simulink library "fmCopterGuidedIndi_lib"  (R2018b)
settings: Solver=VariableStepAuto  StartTime=0.0  StopTime=10.0  RelTol=1e-3
undefined symbols (not defined in the file or in its folder): fm_Traj
libraries: traj_lib x1
settings Model: Creator=Ybeyer  LastModifiedBy=yannic
settings SFSimCC: SimUseLocalCustomCode=off
settings RTWCC: RTWUseLocalCustomCode=off
settings CodeAppCC: StateflowObjectComments=on

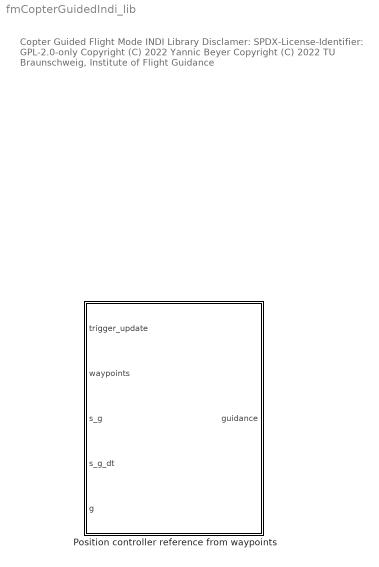
== system fmCopterGuidedIndi_lib ==
  note: Copter Guided Flight Mode INDI Library
      |
      | Disclamer:
      | SPDX-License-Identifier: GPL-2.0-only
      |
      | Copyright (C) 2022 Yannic Beyer
      | Copyright (C) 2022 TU Braunschweig, Institute of Flight Guidance
  Position controller reference from waypoints : Subsystem  mask{fm=fm_Traj, T_inner_loop=0.1}
      mask prompts: fm "Guided flight mode parameters struct, see fmCopterGuidedIndi_params_default"; T_inner_loop "Inner loop time constant seen by position controller, in s"
      mask init:
      | % Create emptry trajectory with a maximum space for 10 waypoints
      | [traj_empty] = trajInit(fm.traj.wpmax, fm.traj.degree);
      | 
      | % Create simulink bus definition
      | assignin('base','trajectoryBus', struct2bus_(traj_empty));
      mask DialogControl DescGroupVar Prompt: Position controller reference from waypoints
      mask DialogControl DescTextVar Prompt: Waypoints are connected by splines. The shortest distance to the desired flight path is computed. Then the corresponding desired position, velocity and acceleration are computed based on the desired flight-path velocity.

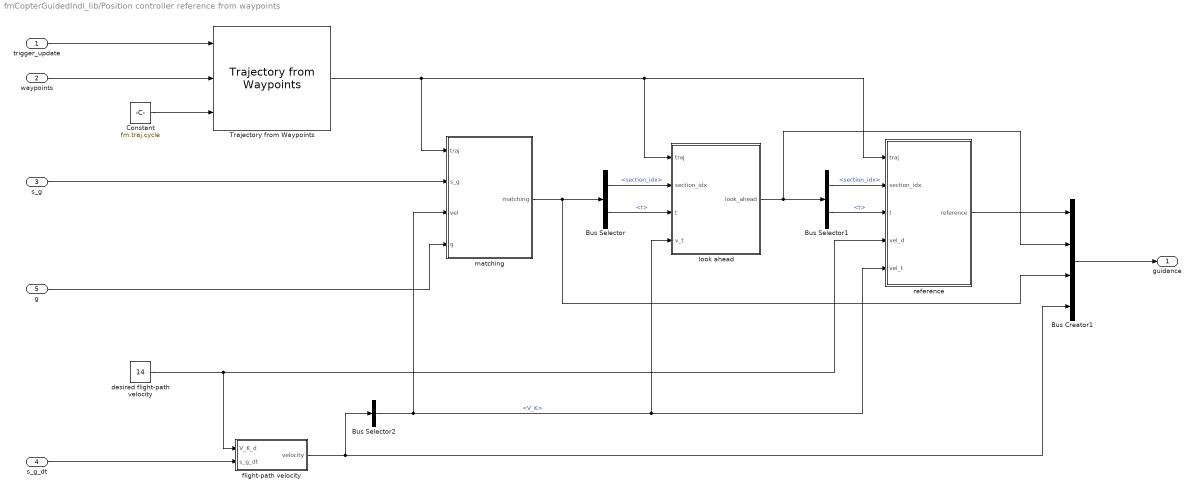
== system fmCopterGuidedIndi_lib/Position controller reference from waypoints ==
  trigger_update : Inport
  waypoints : Inport  Port=2
  s_g : Inport  Port=3
  s_g_dt : Inport  Port=4
  g : Inport  Port=5
  Bus Creator1 : BusCreator  Inputs=4
  Bus Selector : BusSelector  OutputSignals=section_idx,t
  Bus Selector1 : BusSelector  OutputSignals=section_idx,t
  Bus Selector2 : BusSelector  OutputSignals=V_K
  Constant : Constant  Value=fm.traj.cycle
  Trajectory from Waypoints : traj_lib/Trajectory from Waypoints  traj_empty=traj_empty
      settings: SourceProductName=LADAC
  desired flight-path velocity : Constant  Value=14
  flight-path velocity : Subsystem
  look ahead : Subsystem
  matching : Subsystem
  reference : Subsystem
  guidance : Outport
  wires:
  waypoints/1 -> Trajectory from Waypoints/2
  g/1 -> matching/4(g)
  Constant/1 -> Trajectory from Waypoints/3
  trigger_update/1 -> Trajectory from Waypoints/1
  Trajectory from Waypoints/1 -> look ahead/1(traj), reference/1(traj), matching/1(traj)
  s_g/1 -> matching/2(s_g)
  matching/1(matching) -> Bus Creator1/3, Bus Selector/1
  desired flight-path velocity/1 -> flight-path velocity/1(V_K_d), reference/4(vel_d)
  look ahead/1(look_ahead) -> Bus Creator1/2, Bus Selector1/1
  reference/1(reference) -> Bus Creator1/1
  Bus Selector/1 -> look ahead/2(section_idx)  "<section_idx>"
  Bus Selector/2 -> look ahead/3(t)  "<t>"
  Bus Selector1/1 -> reference/2(section_idx)  "<section_idx>"
  Bus Selector1/2 -> reference/3(t)  "<t>"
  Bus Creator1/1 -> guidance/1
  s_g_dt/1 -> flight-path velocity/2(s_g_dt)
  flight-path velocity/1(velocity) -> Bus Creator1/4, Bus Selector2/1
  Bus Selector2/1 -> matching/3(vel), reference/5(vel_t), look ahead/4(v_t)  "<V_K>"

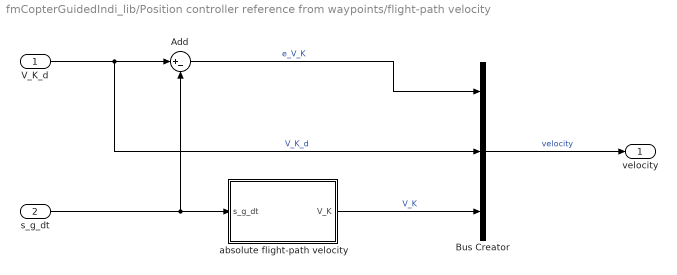
== system fmCopterGuidedIndi_lib/Position controller reference from waypoints/flight-path velocity ==
  V_K_d : Inport
  s_g_dt : Inport  Port=2
  Add : Sum  Inputs=|+-
  Bus Creator : BusCreator  Inputs=3
  absolute flight-path velocity : Subsystem
  velocity : Outport
  wires:
  s_g_dt/1 -> absolute flight-path velocity/1(s_g_dt), Add/2
  absolute flight-path velocity/1(V_K) -> Bus Creator/3  "V_K"
  V_K_d/1 -> Bus Creator/2, Add/1  "V_K_d"
  Bus Creator/1 -> velocity/1  "velocity"
  Add/1 -> Bus Creator/1  "e_V_K"

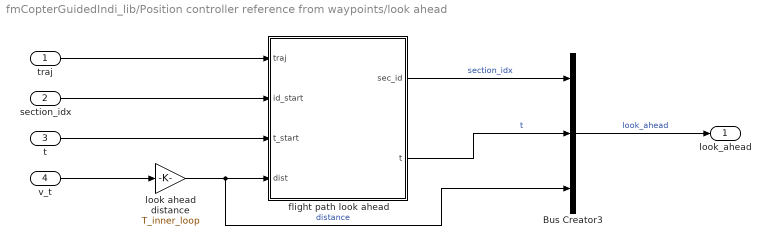
== system fmCopterGuidedIndi_lib/Position controller reference from waypoints/look ahead ==
  traj : Inport
  section_idx : Inport  Port=2
  t : Inport  Port=3
  v_t : Inport  Port=4
  Bus Creator3 : BusCreator  Inputs=3
  flight path look ahead : MATLAB Function  TreatAsAtomicUnit=on
  look ahead distance : Gain  Gain=T_inner_loop
  look_ahead : Outport
  wires:
  v_t/1 -> look ahead distance/1
  flight path look ahead/2(t) -> Bus Creator3/2  "t"
  Bus Creator3/1 -> look_ahead/1  "look_ahead"
  section_idx/1 -> flight path look ahead/2(id_start)
  traj/1 -> flight path look ahead/1(traj)
  flight path look ahead/1(sec_id) -> Bus Creator3/1  "section_idx"
  t/1 -> flight path look ahead/3(t_start)
  look ahead distance/1 -> Bus Creator3/3, flight path look ahead/4(dist)  "distance"

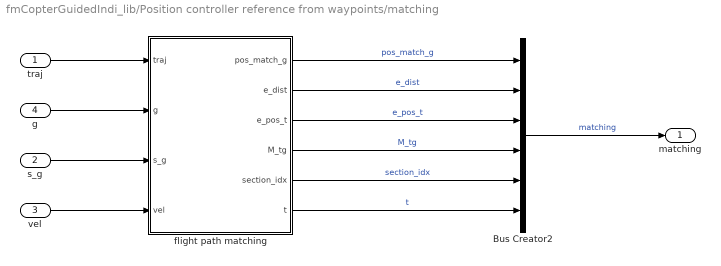
== system fmCopterGuidedIndi_lib/Position controller reference from waypoints/matching ==
  traj : Inport
  s_g : Inport  Port=2
  vel : Inport  Port=3
  g : Inport  Port=4
  Bus Creator2 : BusCreator  Inputs=6
  flight path matching : MATLAB Function  TreatAsAtomicUnit=on
  matching : Outport
  wires:
  flight path matching/5(section_idx) -> Bus Creator2/5  "section_idx"
  traj/1 -> flight path matching/1(traj)
  flight path matching/3(e_pos_t) -> Bus Creator2/3  "e_pos_t"
  flight path matching/6(t) -> Bus Creator2/6  "t"
  g/1 -> flight path matching/2(g)
  flight path matching/1(pos_match_g) -> Bus Creator2/1  "pos_match_g"
  vel/1 -> flight path matching/4(vel)
  flight path matching/2(e_dist) -> Bus Creator2/2  "e_dist"
  s_g/1 -> flight path matching/3(s_g)
  Bus Creator2/1 -> matching/1  "matching"
  flight path matching/4(M_tg) -> Bus Creator2/4  "M_tg"

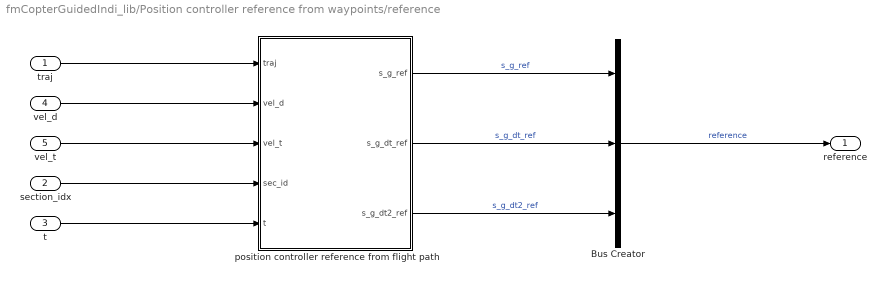
== system fmCopterGuidedIndi_lib/Position controller reference from waypoints/reference ==
  traj : Inport
  section_idx : Inport  Port=2
  t : Inport  Port=3
  vel_d : Inport  Port=4
  vel_t : Inport  Port=5
  Bus Creator : BusCreator  Inputs=3
  position controller reference from flight path : MATLAB Function  TreatAsAtomicUnit=on
  reference : Outport
  wires:
  position controller reference from flight path/1(s_g_ref) -> Bus Creator/1  "s_g_ref"
  vel_d/1 -> position controller reference from flight path/2(vel_d)
  position controller reference from flight path/2(s_g_dt_ref) -> Bus Creator/2  "s_g_dt_ref"
  t/1 -> position controller reference from flight path/5(t)
  position controller reference from flight path/3(s_g_dt2_ref) -> Bus Creator/3  "s_g_dt2_ref"
  traj/1 -> position controller reference from flight path/1(traj)
  Bus Creator/1 -> reference/1  "reference"
  section_idx/1 -> position controller reference from flight path/4(sec_id)
  vel_t/1 -> position controller reference from flight path/3(vel_t)

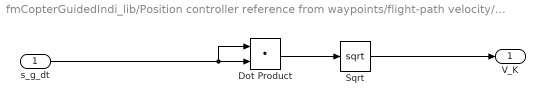
== system fmCopterGuidedIndi_lib/Position controller reference from waypoints/flight-path velocity/absolute flight-path velocity ==
  s_g_dt : Inport
  Dot Product : DotProduct  InputSameDT=on  OutDataTypeStr=Inherit: Inherit via internal rule
  Sqrt : Sqrt  SaturateOnIntegerOverflow=on
  V_K : Outport
  wires:
  Dot Product/1 -> Sqrt/1
  Sqrt/1 -> V_K/1
  s_g_dt/1 -> Dot Product/1, Dot Product/2

== matlab function fmCopterGuidedIndi_lib/Position controller reference from waypoints/reference/position controller reference from flight path ==
  data: traj input; vel_d input; vel_t input; s_g_ref output size=3; s_g_dt_ref output; sec_id input; t input; s_g_dt2_ref output
function [s_g_ref,s_g_dt_ref,s_g_dt2_ref] = fcn(traj, vel_d, vel_t, sec_id, t)
traj_section = trajGetSection(traj,sec_id);
s_g_ref = trajSectionGetPos(traj_section,t);
s_g_dt_ref = trajSectionGetVel(traj_section,vel_d,t);
s_g_dt2_ref = trajSectionGetAcc(traj_section,vel_t,0, t);
end

== matlab function fmCopterGuidedIndi_lib/Position controller reference from waypoints/look ahead/flight path look ahead ==
  data: traj input; sec_id output size=1; id_start input size=1; t_start input; dist input; t output size=1
function [sec_id,t] = trajSweepAlong(traj,id_start,t_start,dist)
[sec_id, t] = trajSweepAlong(traj,id_start,t_start,dist);
end

== matlab function fmCopterGuidedIndi_lib/Position controller reference from waypoints/matching/flight path matching ==
  data: pos_match_g output; e_dist output; e_pos_t output; M_tg output; traj input size=1; section_idx output size=1; g input size=1; s_g input size=3; vel input size=1; t output size=1
function [pos_match_g, e_dist, e_pos_t, M_tg, section_idx, t]  = fcn(traj, g, s_g, vel)

    [section_idx, e_dist, t] = trajGetMatch(traj, s_g);
    
    traj_section   = trajGetSection(traj, section_idx);
    
    pos_match_g = trajSectionGetPos(traj_section,t);
    
    [T, B, N, ~, ~] = trajSectionGetFrenetSerretWithGravity(traj_section, vel, g, t);
    M_tg = [T, B, -N]';
         
    e_pos_t = M_tg * (pos_match_g - s_g);  
    
end
